simulink library "HX_finned_tube_stratified"  (Simulink 7.6)
settings: Solver=ode45  StartTime=0.0  StopTime=10.0  RelTol=1e-3
undefined symbols (not defined in the file): dia, height, nodes
libraries: carnot x2
settings Model: Creator=lena.frank  LastModifiedBy=drhf

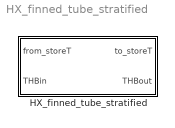
== system HX_finned_tube_stratified ==
  HX_finned_tube_stratified : Subsystem  mask(stratified finned tube heat exchanger for storage){h_in=1, h_out=0, dpipe=0.03, swall=0.002, lpipe=15, cond=50, dfin=0.05, sfin=0.001, nfin=100, dplin=100, dpqua=100, nodes=nodes, hgt=height, dia=dia}
      mask prompts: h_in "relative height of inlet"; h_out "relative height of outlet"; dpipe "outer diameter of HX pipe in m (without fins)"; swall "thickness of pipe wall in m"; lpipe "length of HX pipe in m"; cond "thermal conductivity of HX wall in W/m/K"; dfin "diameter of HX pipe with fins in m"; sfin "wall thickness of fins in m"; nfin "number of fins per length in 1/m"; dplin "pressure drop linear in mdot [Pa*s/kg]"; dpqua "pressure drop quadratic in mdot [Pa*s²/kg²]"; nodes "Number of nodes (DO NOT CHANGE)"; hgt "Height vector (DO NOT CHANGE)"; dia "Diameter (DO NOT CHANGE)"
      mask help:
      | The block transforms the incoming THV vector to a vector which the storage interprets as a heat exchanger.
      | Give inlet and outlet as a relative position 0=bottom to 1=top
      | The heat transfer is calculated by a theoretical equation from Wagner: Waermeuebertragung, Vogel Fachbuch, 1991
      |
      | Stratified:
      | For charging (inlet above outlet) the heat transfer starts when the storage temperature is below the heat exchanger temperature.
      | For discharging (outlet above inlet) the heat transfer starts when the storage temperature is above the heat exchanger temperature.
      mask init:
      | in = zeros(nodes,1);    % vector of length nodes
      | up = in;                % vector of length nodes
      | down = in;              % vector of length nodes
      | 
      | h_in = max(0,h_in);     % no nodes below 0
      | h_out = max(0,h_out);   % no nodes below 0
      | hgt = (h_out-h_in)*hgt;
      | 
      | inlet = round(h_in*(nodes-1))+1;    % inlet position
      | outlet = round(h_out*(nodes-1))+1;  % outlet position
      | 
      | in(inlet)=1;
      | 
      | if (h_in < h_out)           % if inlet below outlet
      |     up(inlet:outlet)=1;     % upwards
      | elseif (h_in > h_out)       % else if inlet above outlet
      |     down(outlet:inlet)=1;   % downwards
      | end
      | 
      | dfin = max(dfin,dpipe);
      | nfin = max(nfin, 0);
      | if (sfin < 1e-5)
      |    sfin = 1e-5;
      |    disp('fin width set to minimum 0.01 mm')
      | end
      mask Help: web(['file:///' fullfile(path_carnot('help'),'StoragePorts_HeatExchangerModels.html')],'-helpbrowser')
      mask TabNameString: Heat Exchanger,Heat Exchanger,Heat Exchanger,Heat Exchanger,Heat Exchanger,Heat Exchanger,Heat Exchanger,Heat Exchanger,Heat Exchanger,Pressure drop,Pressure drop,Top mask parameters,Top mask parameters,Top mask parameters
      mask Display: disp('HX finned tube STRAT')

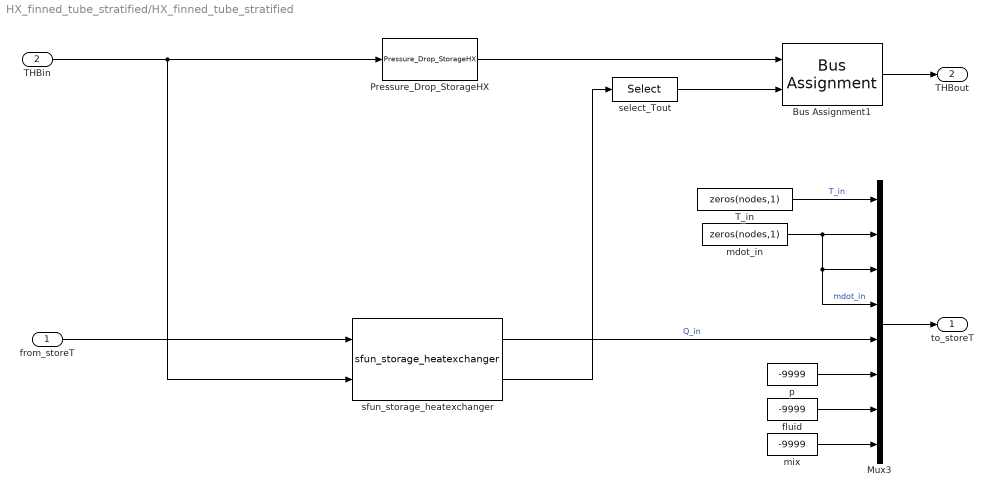
== system HX_finned_tube_stratified/HX_finned_tube_stratified ==
  from_storeT : Inport
  THBin : Inport  Port=2
  Bus Assignment1 : BusAssignment  AssignedSignals=Temperature
  Mux3 : Mux  Inputs=8
  Pressure_Drop_StorageHX : carnot/Basic/Pressure_Drop/Pressure_Drop_StorageHX  SystemSampleTime=-1  dia=dia  hgt=hgt
  T_in : Constant  Value=zeros(nodes,1)
  fluid : Constant  Value=-9999
  mdot_in : Constant  Value=zeros(nodes,1)
  mix : Constant  Value=-9999
  p : Constant  Value=-9999
  select_Tout : Selector  InputPortWidth=nodes  IndexOptions=Index vector (dialog)  Indices=[outlet]  OutputSizes=1
  sfun_storage_heatexchanger : carnot/Basic/Thermal_Models/sfun_storage_heatexchanger  SystemSampleTime=-1  idn="finned tube theoretical  - stratified"  nodes=nodes  inlet=inlet  outlet=outlet  pp=[dpipe, swall, lpipe, cond, dfin, sfin, nfin]
  to_storeT : Outport  InitialOutput=0
  THBout : Outport  Port=2  InitialOutput=0
  wires:
  from_storeT/1 -> sfun_storage_heatexchanger/1
  THBin/1 -> Pressure_Drop_StorageHX/1, sfun_storage_heatexchanger/2
  mdot_in/1 -> Mux3/2, Mux3/3, Mux3/4  "mdot_in"
  Mux3/1 -> to_storeT/1
  select_Tout/1 -> Bus Assignment1/2
  T_in/1 -> Mux3/1  "T_in"
  sfun_storage_heatexchanger/1 -> Mux3/5  "Q_in"
  Bus Assignment1/1 -> THBout/1
  p/1 -> Mux3/6
  fluid/1 -> Mux3/7
  mix/1 -> Mux3/8
  sfun_storage_heatexchanger/2 -> select_Tout/1
  Pressure_Drop_StorageHX/1 -> Bus Assignment1/1
